simulink model "HW2_Simulation_R2021b"  (R2021b)
settings: Solver=FixedStepAuto  StartTime=0.0  StopTime=8  FixedStep=1e-5  MaxStep=1e-5  RelTol=1e-3
model workspace (MAT data in the model file):
  B = 0
  J = 0.068
  Ka = 1
  Ki1 = 155.019969444
  Ki2 = 50
  Kp1 = 1.1884864324
  Kp2 = 3.4
  La = 0.0023
  Lf = 1.44
  M = 1.304
  Ra = 0.3
  Rf = 356.7
  fsw = 10000
  ia_rated = 27
  s = tf
  s.IOSize_ = [1 1]
  s.Data_ = ltipack.tfdata
  s.Data_.num = {[1 0]}
  s.Data_.den = {[0 1]}
  s.Data_.Delay.Input = 0
  s.Data_.Delay.Output = 0
  s.Data_.Delay.IO = 0
  s.Data_.Ts = 0
  vt_rated = 230
  w1 = 500
  w2 = 50
  wbase = 261.799387799
undefined symbols (not defined in the file): DiscIntNeverNeededParam, irated_dq, sigbuilder_block
libraries: simulink x2
settings Model: Creator=EE_CU  LastModifiedBy=surapong
settings SolverCC: AlgebraicLoopSolver=TrustRegion
settings DataIOCC: SaveFormat=Array  ReturnWorkspaceOutputs=off
settings OptimizationCC: BlockReduction=off  BooleanDataType=off
settings DebuggingCC: SaveWithParameterizedLinksMsg=none  UnderspecifiedInitializationDetection=Classic  MergeDetectMultiDrivingBlocksExec=none  SignalResolutionControl=TryResolveAllWithWarning  InheritedTsInSrcMsg=none  MultiTaskDSMMsg=warning  MultiTaskCondExecSysMsg=none  UnconnectedInputMsg=none  UnconnectedOutputMsg=none  UnconnectedLineMsg=none  SFMachineParentedDataDiag=warning
settings HardwareCC: TargetUnknown=on
settings ModelReferenceCC: PropagateSignalLabelsOutOfModel=off
settings SFSimCC: CustomCodeUndefinedFunction=UseInterfaceOnly

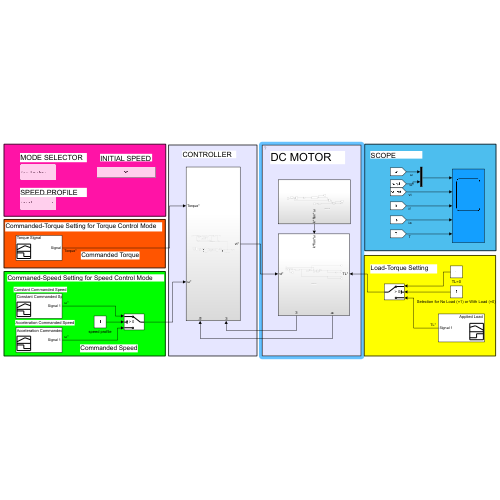
[thumbnail: Simulink's stored preview of the top-level diagram]
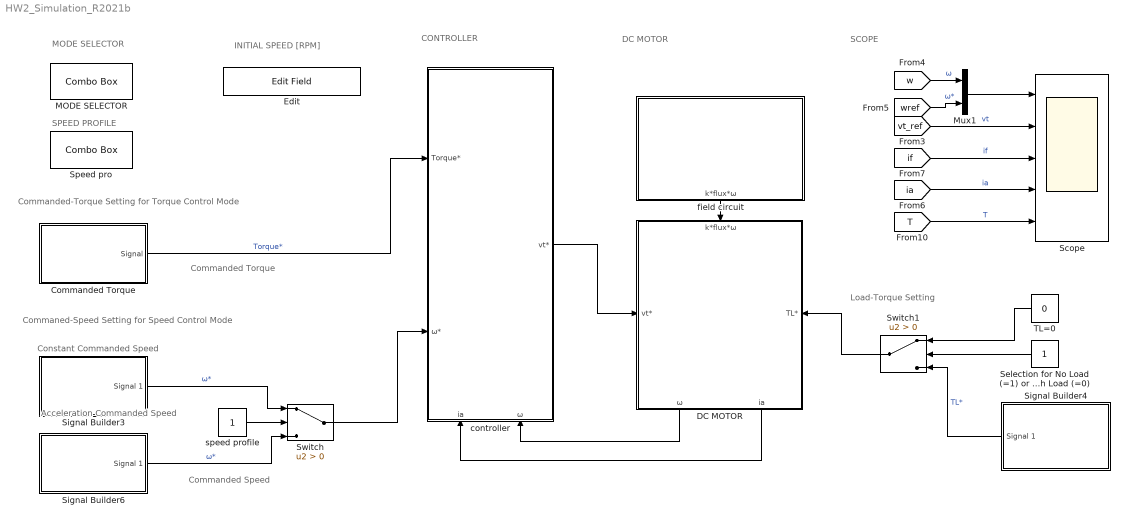
== system HW2_Simulation_R2021b ==
  note: Commanded Torque
  note: Constant Commanded Speed
  note: MODE SELECTOR
  note: Acceleration Commanded Speed
  note: INITIAL SPEED [RPM]
  note: SPEED PROFILE
  note: Commanded-Torque Setting for Torque Control Mode
  note: Commaned-Speed Setting for Speed Control Mode
  note: Load-Torque Setting
  note: SCOPE
  note: DC MOTOR
  note: CONTROLLER
  note: Commanded Speed
  Commanded Torque : Subsystem  Tag=STV Subsys  LoadFcn=sigbuilder_block('load');  StartFcn=sigbuilder_block('start');  StopFcn=sigbuilder_block('stop');  ClipboardFcn=sigbuilder_block('clipboard');  mask(Sigbuilder block){tuvar=[0:10]}
      mask help: Simulink:masks:SigbuilderBlock_MD
      mask init:
      | if ~strcmp(get_param(bdroot(gcbh),'SimulationStatus'),'stopped') tuvar = sigbuilder_block('maskInit'); end
      settings: CopyFcn=sigbuilder_block('copy');  DeleteFcn=sigbuilder_block('delete');  ModelCloseFcn=sigbuilder_block('modelClose');  PreSaveFcn=sigbuilder_block('preSave');  PauseFcn=sigbuilder_block('pause');  ContinueFcn=sigbuilder_block('continue');  NameChangeFcn=sigbuilder_block('namechange');  OpenFcn=sigbuilder_block('open',[5.5 30 949 418 ]);  CloseFcn=sigbuilder_block('close');
      mask Display: plot(0, 0, 100, 100,[2, 2, 32, 32, 2], [68, 8, 8, 68, 68],[32, 2], [38, 38], [32, 19, 2],[53, 60, 44], [32, 17, 17, 2],[16, 16, 31, 31]);txt = getActiveGroup(gcbh);text(2, 100, txt,'verticalAlignment', 'top');
  DC MOTOR : Subsystem
      settings: PortSchema="{\"entries\":[{\"content\":{\"sides\":[{\"content\":{\"connectorIds\":[\"In1\"]},\"type\":\"ConnectorPlacement.EquallySpacedRectSide\",\"uuid\":\"a5d9886d-da64-4ef1-a5a6-c78ada3bfc19\"},{\"content\":{\"connectorIds\":[\"In3\"],\"side\":\"RIGHT\"},\"type\":\"ConnectorPlacement.EquallySpacedRectSide\",\"uuid\":\"368b0381-86ca-4eec-8726-91c10a4720dc\"},{\"content\":{\"connectorIds\":[\"In2\"],\"side\":\"TOP\"},\"type\":\"ConnectorPlacement.EquallySpacedRectSide\",\"uuid\":\"413bc0da-9218-4534-b65b-355027a9209b\"},{\"content\":{\"connectorIds\":[\"Out1\",\"Out2\"],\"side\":\"BOTTOM\"},\"type\":\"ConnectorPlacement.EquallySpacedRectSide\",\"uuid\":\"37857b30-64cf-45fe-8840-7abacb4e931c\"}]},\"type\":\"ConnectorPlacement.EquallySpacedConnector\",\"uuid\":\"fbdb1576-573e-44b8-b639-49e1df1499a9\"}],\"packageUris\":[\"http://schema.mathworks.com/mf0/Connector/R2020b\"],\"version\":\"1.0\"}"
  Edit : EditField  LabelPosition=Hide  ShowInitialText=on  Alignment=Center
  MODE SELECTOR : ComboBox  LabelPosition=Hide  SelectedLabel=Speed-Control Mode
      settings: Values={{'Torque-Control Mode', 'Speed-Control Mode'}, [0 1]}
  Mux1 : Mux  Inputs=2
  Scope : Scope  NumInputPorts=5
  Selection for No Load (=1) or With Load (=0) : Constant
  Signal Builder3 : Subsystem  Tag=STV Subsys  LoadFcn=sigbuilder_block('load');  StartFcn=sigbuilder_block('start');  StopFcn=sigbuilder_block('stop');  ClipboardFcn=sigbuilder_block('clipboard');  mask(Sigbuilder block){tuvar=[0:10]}
      mask help: Simulink:masks:SigbuilderBlock_MD
      mask init:
      | if ~strcmp(get_param(bdroot(gcbh),'SimulationStatus'),'stopped') tuvar = sigbuilder_block('maskInit'); end
      settings: CopyFcn=sigbuilder_block('copy');  DeleteFcn=sigbuilder_block('delete');  ModelCloseFcn=sigbuilder_block('modelClose');  PreSaveFcn=sigbuilder_block('preSave');  PauseFcn=sigbuilder_block('pause');  ContinueFcn=sigbuilder_block('continue');  NameChangeFcn=sigbuilder_block('namechange');  OpenFcn=sigbuilder_block('open',[5.5 30 949 418 ]);  CloseFcn=sigbuilder_block('close');
      mask Display: plot(0, 0, 100, 100,[2, 2, 32, 32, 2], [68, 8, 8, 68, 68],[32, 2], [38, 38], [32, 19, 2],[53, 60, 44], [32, 17, 17, 2],[16, 16, 31, 31]);txt = getActiveGroup(gcbh);text(2, 100, txt,'verticalAlignment', 'top');
  Signal Builder4 : Subsystem  Tag=STV Subsys  LoadFcn=sigbuilder_block('load');  StartFcn=sigbuilder_block('start');  StopFcn=sigbuilder_block('stop');  ClipboardFcn=sigbuilder_block('clipboard');  mask(Sigbuilder block){tuvar=[0:10]}
      mask help: Simulink:masks:SigbuilderBlock_MD
      mask init:
      | if ~strcmp(get_param(bdroot(gcbh),'SimulationStatus'),'stopped') tuvar = sigbuilder_block('maskInit'); end
      settings: CopyFcn=sigbuilder_block('copy');  DeleteFcn=sigbuilder_block('delete');  ModelCloseFcn=sigbuilder_block('modelClose');  PreSaveFcn=sigbuilder_block('preSave');  PauseFcn=sigbuilder_block('pause');  ContinueFcn=sigbuilder_block('continue');  NameChangeFcn=sigbuilder_block('namechange');  OpenFcn=sigbuilder_block('open',[5.5 30 949 418 ]);  CloseFcn=sigbuilder_block('close');
      mask Display: plot(0, 0, 100, 100,[2, 2, 32, 32, 2], [68, 8, 8, 68, 68],[32, 2], [38, 38], [32, 19, 2],[53, 60, 44], [32, 17, 17, 2],[16, 16, 31, 31]);txt = getActiveGroup(gcbh);text(2, 100, txt,'verticalAlignment', 'top');
  Signal Builder6 : Subsystem  Tag=STV Subsys  LoadFcn=sigbuilder_block('load');  StartFcn=sigbuilder_block('start');  StopFcn=sigbuilder_block('stop');  ClipboardFcn=sigbuilder_block('clipboard');  mask(Sigbuilder block){tuvar=[0:10]}
      mask help: Simulink:masks:SigbuilderBlock_MD
      mask init:
      | if ~strcmp(get_param(bdroot(gcbh),'SimulationStatus'),'stopped') tuvar = sigbuilder_block('maskInit'); end
      settings: CopyFcn=sigbuilder_block('copy');  DeleteFcn=sigbuilder_block('delete');  ModelCloseFcn=sigbuilder_block('modelClose');  PreSaveFcn=sigbuilder_block('preSave');  PauseFcn=sigbuilder_block('pause');  ContinueFcn=sigbuilder_block('continue');  NameChangeFcn=sigbuilder_block('namechange');  OpenFcn=sigbuilder_block('open',[5.5 30 949 418 ]);  CloseFcn=sigbuilder_block('close');
      mask Display: plot(0, 0, 100, 100,[2, 2, 32, 32, 2], [68, 8, 8, 68, 68],[32, 2], [38, 38], [32, 19, 2],[53, 60, 44], [32, 17, 17, 2],[16, 16, 31, 31]);txt = getActiveGroup(gcbh);text(2, 100, txt,'verticalAlignment', 'top');
  Speed pro : ComboBox  LabelPosition=Hide  SelectedLabel=Constant
      settings: Values={{'Constant', 'Acceleration'}, [1 0]}
  Switch : Switch  Criteria=u2 > Threshold
  Switch1 : Switch  Criteria=u2 > Threshold
  TL=0 : Constant  Value=0
  controller : Subsystem
      settings: PortSchema="{\"entries\":[{\"content\":{\"sides\":[{\"content\":{\"connectorIds\":[\"In1\",\"In2\"]},\"type\":\"ConnectorPlacement.EquallySpacedRectSide\",\"uuid\":\"4203f81f-4d91-40d7-be1b-89a545b9c722\"},{\"content\":{\"connectorIds\":[\"Out1\"],\"side\":\"RIGHT\"},\"type\":\"ConnectorPlacement.EquallySpacedRectSide\",\"uuid\":\"d697897f-ff4c-47d6-92e8-8b3e50432737\"},{\"content\":{\"connectorIds\":[],\"side\":\"TOP\"},\"type\":\"ConnectorPlacement.EquallySpacedRectSide\",\"uuid\":\"e5ba2846-a1ea-4dd1-aab0-295b901491f7\"},{\"content\":{\"connectorIds\":[\"In3\",\"In4\"],\"side\":\"BOTTOM\"},\"type\":\"ConnectorPlacement.EquallySpacedRectSide\",\"uuid\":\"f1006170-3159-4a4b-856d-a8f1959ce5c6\"}]},\"type\":\"ConnectorPlacement.EquallySpacedConnector\",\"uuid\":\"6d817abf-3150-42c3-91f7-71efc1a1c1e5\"}],\"packageUris\":[\"http://schema.mathworks.com/mf0/Connector/R2020b\"],\"version\":\"1.0\"}"
  field circuit : Subsystem
  speed profile : Constant
  wires:
  controller/1(vt*) -> DC MOTOR/1(vt*)
  DC MOTOR/1(ω) -> controller/4(ω)
  [w] -> Mux1/1  "ω"
  [wref] -> Mux1/2  "ω*"
  Commanded Torque/1(Signal) -> controller/1(Torque*)  "Torque*"
  field circuit/1(k*flux*ω) -> DC MOTOR/2(k*flux*ω)
  Signal Builder3/1(Signal 1) -> Switch/1  "ω*"
  Signal Builder6/1(Signal 1) -> Switch/3  "ω*"
  speed profile/1 -> Switch/2
  Mux1/1 -> Scope/1
  [if] -> Scope/3  "if"
  [T] -> Scope/5  "T"
  [vt_ref] -> Scope/2  "vt"
  DC MOTOR/2(ia) -> controller/3(ia)
  [ia] -> Scope/4  "ia"
  Switch/1 -> controller/2(ω*)
  Switch1/1 -> DC MOTOR/3(TL*)
  Signal Builder4/1(Signal 1) -> Switch1/3  "TL*"
  Selection for No Load (=1) or With Load (=0)/1 -> Switch1/2
  TL=0/1 -> Switch1/1

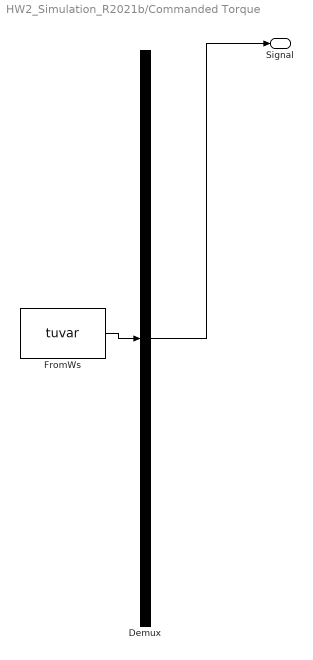
== system HW2_Simulation_R2021b/Commanded Torque ==
  Demux : Demux  Tag=STV Demux  Outputs=1
      settings: DisplayOption=none
  FromWs : FromWorkspace  Tag=STV FromWs  VariableName=tuvar
      SigBuilderData=|
      | common.afterFinalStr = 'Extrapolate'
      | common.sampleTime = 0
      | dataSet.timeRange = [0 8]
      | dataSet.name = 'Torque Signal'
      | sbobj.Groups.Name = 'Torque Signal'
      | sbobj.Groups.Signals.Name = 'Signal'
      | sbobj.Groups.Signals.XData = [0 1 2 3 5.01 6 7 8]
      | sbobj.Groups.Signals.YData = [0 0 0 0 0 0 0 0]
      | sbobj.Groups.TimeRange = [0 8]
  Signal : Outport  Tag=STV Outport
  wires:
  Demux/1 -> Signal/1
  FromWs/1 -> Demux/1

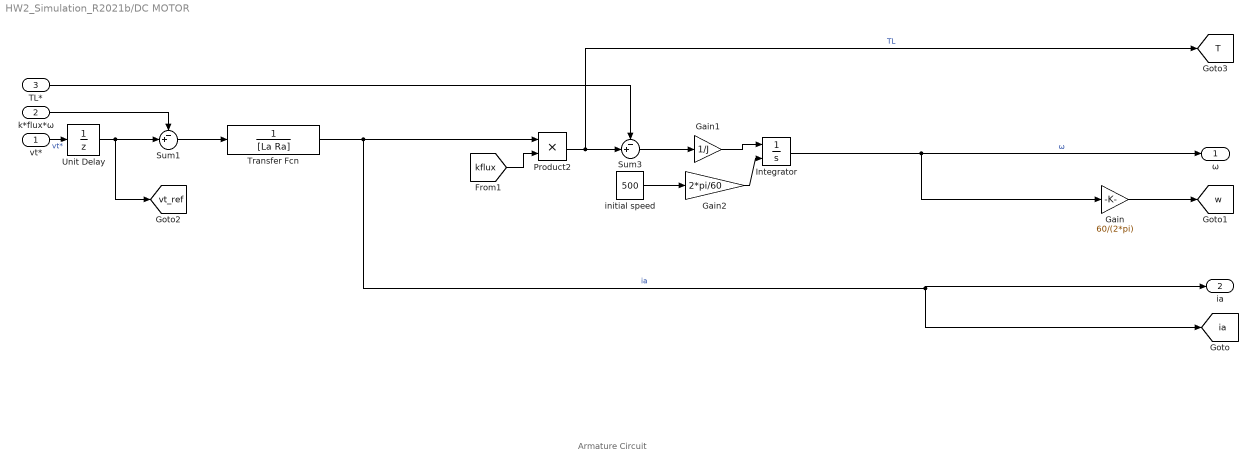
== system HW2_Simulation_R2021b/DC MOTOR ==
  note: Armature Circuit
  vt* : Inport
  k*flux*ω : Inport  Port=2
  TL* : Inport  Port=3
  Gain : Gain  Gain=60/(2*pi)
  Gain1 : Gain  Gain=1/J
  Gain2 : Gain  Gain=2*pi/60
  Integrator : Integrator  InitialConditionSource=external  InitialCondition=500*2*pi/60
  Product2 : Product
  Sum1 : Sum  Inputs=-+|
  Sum3 : Sum  Inputs=-+|
  Transfer Fcn : TransferFcn  Denominator=[La Ra]
  Unit Delay : UnitDelay  SampleTime=-1  HasFrameUpgradeWarning=on
  initial speed : Constant  Value=500
  ω : Outport
  ia : Outport  Port=2
  tag scope: T=global, ia=global, vt_ref=global, w=global
  wires:
  Sum1/1 -> Transfer Fcn/1
  Transfer Fcn/1 -> [ia], ia/1, Product2/1  "ia"
  Product2/1 -> [T], Sum3/2  "TL"
  [kflux] -> Product2/2
  TL*/1 -> Sum3/1
  Integrator/1 -> Gain/1, ω/1  "ω"
  k*flux*ω/1 -> Sum1/1
  vt*/1 -> Unit Delay/1  "vt*"
  Gain/1 -> [w]
  Gain1/1 -> Integrator/1
  initial speed/1 -> Gain2/1
  Gain2/1 -> Integrator/2
  Sum3/1 -> Gain1/1
  Unit Delay/1 -> [vt_ref], Sum1/2

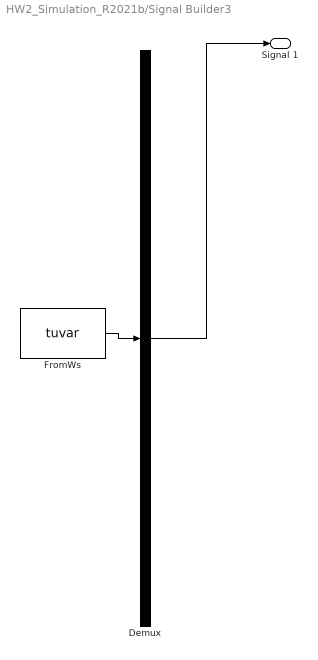
== system HW2_Simulation_R2021b/Signal Builder3 ==
  Demux : Demux  Tag=STV Demux  Outputs=1
      settings: DisplayOption=none
  FromWs : FromWorkspace  Tag=STV FromWs  VariableName=tuvar
      SigBuilderData=|
      | common.afterFinalStr = 'Extrapolate'
      | common.sampleTime = 0
      | dataSet.timeRange = [0 12]
      | dataSet.name = 'Constant Commanded Speed'
      | sbobj.Groups.Name = 'Constant Commanded Speed'
      | sbobj.Groups.Signals.Name = 'Signal 1'
      | sbobj.Groups.Signals.XData = [0 1.01 3 12]
      | sbobj.Groups.Signals.YData = [2000 2000 2000 2000]
      | sbobj.Groups.TimeRange = [0 12]
  Signal 1 : Outport  Tag=STV Outport
  wires:
  FromWs/1 -> Demux/1
  Demux/1 -> Signal 1/1

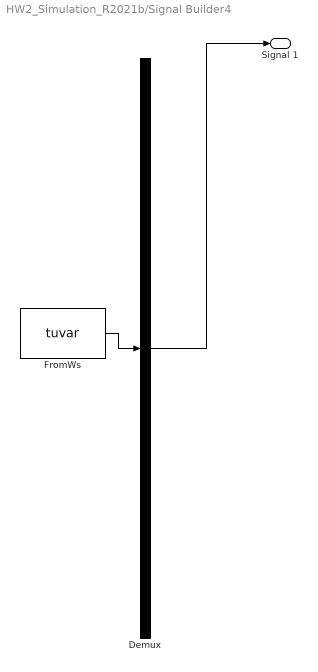
== system HW2_Simulation_R2021b/Signal Builder4 ==
  Demux : Demux  Tag=STV Demux  Outputs=1
      settings: DisplayOption=none
  FromWs : FromWorkspace  Tag=STV FromWs  VariableName=tuvar
      SigBuilderData=|
      | common.afterFinalStr = 'Extrapolate'
      | common.sampleTime = 0
      | dataSet.timeRange = [0 8]
      | dataSet.name = 'Applied Load'
      | sbobj.Groups.Name = 'Applied Load'
      | sbobj.Groups.Signals.Name = 'Signal 1'
      | sbobj.Groups.Signals.XData = [0 3 3 8]
      | sbobj.Groups.Signals.YData = [0 0 15 15]
      | sbobj.Groups.TimeRange = [0 8]
  Signal 1 : Outport  Tag=STV Outport
  wires:
  FromWs/1 -> Demux/1
  Demux/1 -> Signal 1/1

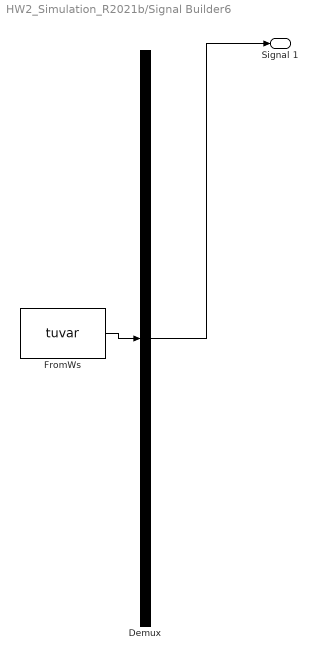
== system HW2_Simulation_R2021b/Signal Builder6 ==
  Demux : Demux  Tag=STV Demux  Outputs=1
      settings: DisplayOption=none
  FromWs : FromWorkspace  Tag=STV FromWs  VariableName=tuvar
      SigBuilderData=|
      | common.afterFinalStr = 'Extrapolate'
      | common.sampleTime = 0
      | dataSet.timeRange = [0 4]
      | dataSet.name = 'Acceleration Commanded Speed'
      | sbobj.Groups.Name = 'Acceleration Commanded Speed'
      | sbobj.Groups.Signals.Name = 'Signal 1'
      | sbobj.Groups.Signals.XData = [0 1 1.8 4]
      | sbobj.Groups.Signals.YData = [500 500 4500 4500]
      | sbobj.Groups.TimeRange = [0 4]
  Signal 1 : Outport  Tag=STV Outport
  wires:
  Demux/1 -> Signal 1/1
  FromWs/1 -> Demux/1

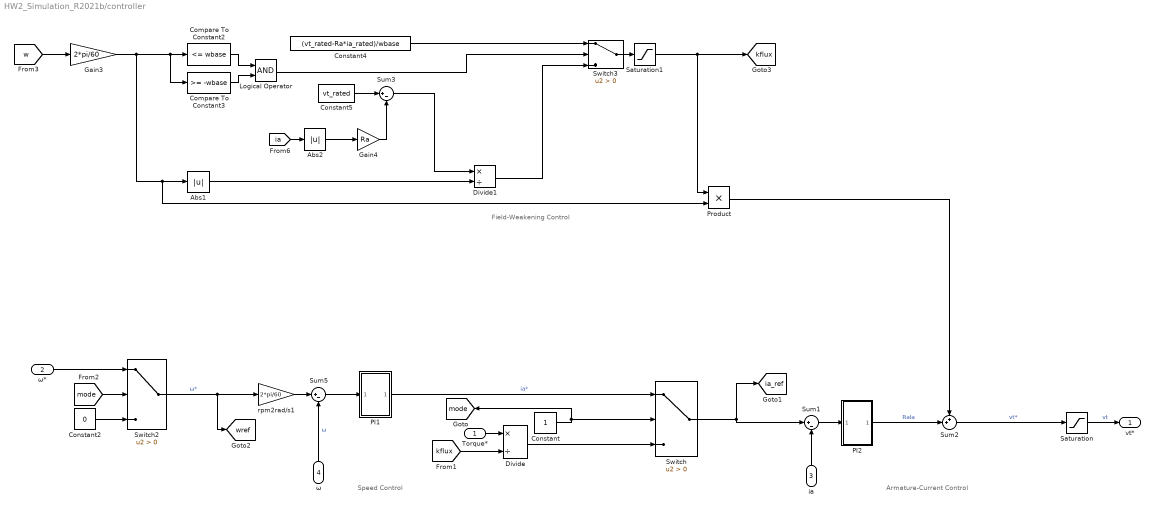
== system HW2_Simulation_R2021b/controller ==
  note: Armature-Current Control
  note: Field-Weakening Control
  note: Speed Control
  Torque* : Inport
  ω* : Inport  Port=2
  ia : Inport  Port=3
  ω : Inport  Port=4
  Abs1 : Abs
  Abs2 : Abs
  Compare To Constant2 : simulink/Logic and Bit Operations/Compare To Constant  relop=<=  const=wbase  OutDataTypeStr=boolean
  Compare To Constant3 : simulink/Logic and Bit Operations/Compare To Constant  relop=>=  const=-wbase  OutDataTypeStr=boolean
  Constant : Constant
  Constant2 : Constant  Value=0
  Constant4 : Constant  Value=(vt_rated-Ra*ia_rated)/wbase
  Constant5 : Constant  Value=vt_rated
  Divide : Product  Inputs=*/
  Divide1 : Product  Inputs=*/
  Gain3 : Gain  Gain=2*pi/60
  Gain4 : Gain  Gain=Ra
  Logical Operator : Logic  AllPortsSameDT=off  OutDataTypeStr=boolean
  PI1 : Subsystem  mask{Kp=Kp2, Ki=Ki2, uplim=27, lolim=-27, Ti=1/w2}
      mask prompts: uplim "Upper Limit"; lolim "Lower Limit"
  PI2 : Subsystem  mask{Kp=Kp1, Ki=Ki1, uplim=inf, lolim=-inf, Ti=1/w1}
      mask prompts: uplim "Upper Limit"; lolim "Lower Limit"
  Product : Product
  Saturation : Saturate  UpperLimit=240  LowerLimit=-240
  Saturation1 : Saturate  UpperLimit=inf  LowerLimit=0.2
  Sum1 : Sum  Inputs=|+-
  Sum2 : Sum  Inputs=++|
  Sum3 : Sum  Inputs=|+-
  Sum5 : Sum  Inputs=|+-
  Switch : Switch  Criteria=u2 > Threshold
  Switch2 : Switch  Criteria=u2 > Threshold
  Switch3 : Switch  Criteria=u2 > Threshold
  rpm2rad/s1 : Gain  Gain=2*pi/60
  vt* : Outport
  tag scope: ia_ref=global, kflux=global, mode=global, wref=global
  wires:
  PI2/1(Out2) -> Sum2/2  "RaIa"
  Sum5/1 -> PI1/1(In2)
  Sum2/1 -> Saturation/1  "vt*"
  PI1/1(Out2) -> Switch/1  "ia*"
  Saturation/1 -> vt*/1  "vt"
  Constant/1 -> [mode], Switch/2
  Torque*/1 -> Divide/1
  [kflux] -> Divide/2
  Sum1/1 -> PI2/1(In2)
  ia/1 -> Sum1/2
  Switch/1 -> Sum1/1, [ia_ref]
  ω/1 -> Sum5/2  "ω"
  Divide/1 -> Switch/3
  ω*/1 -> Switch2/1
  [mode] -> Switch2/2
  Constant2/1 -> Switch2/3
  Switch2/1 -> [wref], rpm2rad/s1/1  "ω*"
  rpm2rad/s1/1 -> Sum5/1
  Switch3/1 -> Saturation1/1
  Product/1 -> Sum2/1
  Constant4/1 -> Switch3/1
  Gain3/1 -> Compare To Constant3/1, Compare To Constant2/1, Product/2, Abs1/1
  Constant5/1 -> Sum3/1
  Sum3/1 -> Divide1/1
  Gain4/1 -> Sum3/2
  Divide1/1 -> Switch3/3
  Compare To Constant2/1 -> Logical Operator/1
  Compare To Constant3/1 -> Logical Operator/2
  Logical Operator/1 -> Switch3/2
  Abs1/1 -> Divide1/2
  [w] -> Gain3/1
  Abs2/1 -> Gain4/1
  [ia] -> Abs2/1
  Saturation1/1 -> Product/1, [kflux]

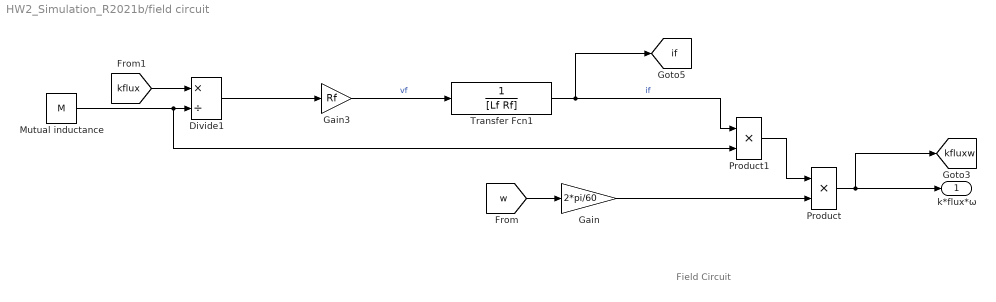
== system HW2_Simulation_R2021b/field circuit ==
  note: Field Circuit
  Divide1 : Product  Inputs=*/
  Gain : Gain  Gain=2*pi/60
  Gain3 : Gain  Gain=Rf
  Mutual inductance : Constant  Value=M
  Product : Product
  Product1 : Product
  Transfer Fcn1 : TransferFcn  Denominator=[Lf Rf]
  k*flux*ω : Outport
  tag scope: if=global, kfluxw=global
  wires:
  Divide1/1 -> Gain3/1
  Product/1 -> k*flux*ω/1, [kfluxw]
  [w] -> Gain/1
  Gain/1 -> Product/2
  Gain3/1 -> Transfer Fcn1/1  "vf"
  Transfer Fcn1/1 -> [if], Product1/1  "if"
  Mutual inductance/1 -> Product1/2, Divide1/2
  Product1/1 -> Product/1
  [kflux] -> Divide1/1

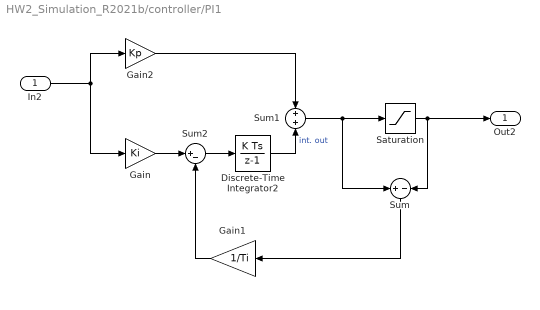
== system HW2_Simulation_R2021b/controller/PI1 ==
  In2 : Inport
  Discrete-Time Integrator2 : DiscreteIntegrator  gainval=1  SampleTime=-1  UpperSaturationLimit=1.2*irated_dq  LowerSaturationLimit=-1.2*irated_dq  ICPrevOutput=DiscIntNeverNeededParam  ICPrevScaledInput=DiscIntNeverNeededParam
  Gain : Gain  Gain=Ki
  Gain1 : Gain  Gain=1/Ti
  Gain2 : Gain  Gain=Kp
  Saturation : Saturate  UpperLimit=uplim  LowerLimit=lolim
  Sum : Sum  Inputs=+-
  Sum1 : Sum
  Sum2 : Sum  Inputs=|+-
  Out2 : Outport
  wires:
  Gain1/1 -> Sum2/2
  Sum/1 -> Gain1/1
  Gain/1 -> Sum2/1
  Sum2/1 -> Discrete-Time Integrator2/1
  Discrete-Time Integrator2/1 -> Sum1/2  "int. out"
  Gain2/1 -> Sum1/1
  In2/1 -> Gain2/1, Gain/1
  Sum1/1 -> Sum/1, Saturation/1
  Saturation/1 -> Out2/1, Sum/2

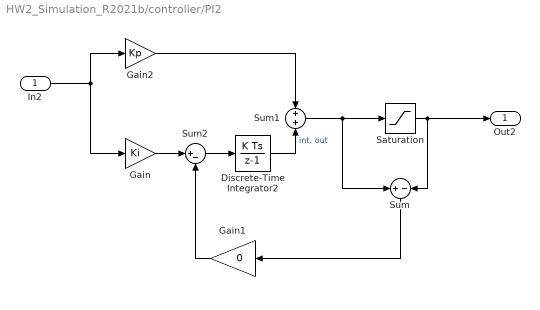
== system HW2_Simulation_R2021b/controller/PI2 ==
  In2 : Inport
  Discrete-Time Integrator2 : DiscreteIntegrator  gainval=1  InitialCondition=0.00001  SampleTime=-1  UpperSaturationLimit=1.2*irated_dq  LowerSaturationLimit=-1.2*irated_dq  ICPrevOutput=DiscIntNeverNeededParam  ICPrevScaledInput=DiscIntNeverNeededParam
  Gain : Gain  Gain=Ki
  Gain1 : Gain  Gain=0
  Gain2 : Gain  Gain=Kp
  Saturation : Saturate  UpperLimit=uplim  LowerLimit=lolim
  Sum : Sum  Inputs=+-
  Sum1 : Sum
  Sum2 : Sum  Inputs=|+-
  Out2 : Outport
  wires:
  Saturation/1 -> Sum/2, Out2/1
  Sum1/1 -> Saturation/1, Sum/1
  In2/1 -> Gain/1, Gain2/1
  Gain2/1 -> Sum1/1
  Discrete-Time Integrator2/1 -> Sum1/2  "int. out"
  Sum2/1 -> Discrete-Time Integrator2/1
  Gain/1 -> Sum2/1
  Sum/1 -> Gain1/1
  Gain1/1 -> Sum2/2
